simulink model "simulacija"  (Simulink 10.2)
settings: Solver=ode45  StartTime=0.0  StopTime=150  RelTol=1e-3
libraries: simulink x3, fuzblock x1
settings Model: Creator=Aleksandar Markovic  LastModifiedBy=zelimir
settings DataIOCC: SaveFormat=StructureWithTime  SignalLoggingSaveFormat=Dataset
settings DebuggingCC: UnderspecifiedInitializationDetection=Simplified  MergeDetectMultiDrivingBlocksExec=error  SFUnexpectedBacktrackingDiag=error  SFNoUnconditionalDefaultTransitionDiag=error
settings HardwareCC: ProdBitPerPointer=64  ProdLargestAtomicFloat=Float  ProdIntDivRoundTo=Zero  ProdEndianess=LittleEndian  ProdHWDeviceType=Specified
settings GRTTargetCC: TargetLangStandard=C99 (ISO)
settings ConfigComp: CovMetricSettings=dwe  CovSaveCumulativeToWorkspaceVar=off  CovSaveSingleToWorkspaceVar=off  CovExternalEMLEnable=on

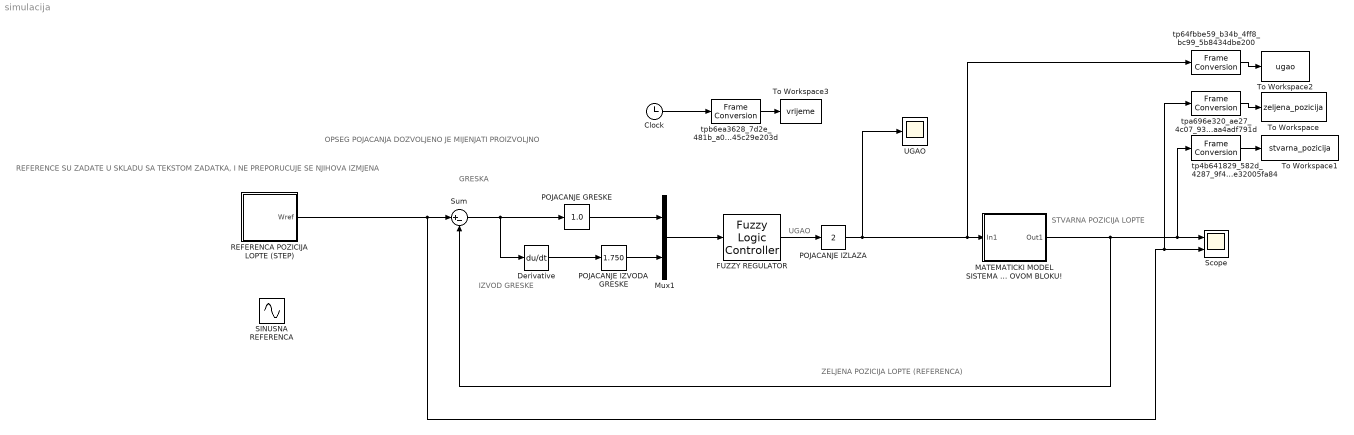
== system simulacija ==
  note: REFERENCE SU ZADATE U SKLADU SA TEKSTOM ZADATKA, I NE PREPORUCUJE SE NJIHOVA IZMJENA
  note: OPSEG POJACANJA DOZVOLJENO JE MIJENJATI PROIZVOLJNO
  note: ZELJENA POZICIJA LOPTE (REFERENCA)
  note: UGAO
  note: GRESKA
  note: IZVOD GRESKE
  note: STVARNA POZICIJA LOPTE
  Clock : Clock
  Derivative : Derivative
  FUZZY REGULATOR : fuzblock/Fuzzy Logic  Controller  FIS='Regulator.fis'  OutputSampleNumber=101  DataType=double  FuzzifiedInputs=off  RuleFiringStrengths=off  RuleOutputs=off  AggregatedOutputs=off  SimulateUsing=Interpreted execution  OutOfRangeInputValueMessage=warning  NoRuleFiredMessage=warning  EmptyOutputFuzzySetMessage=warning
  "MATEMATICKI MODEL SISTEMA OSIM POCETNE POZICIJE,  NE MIJENJATI NISTA DRUGO U OVOM BLOKU!" : Subsystem  mask{pocetna_pozicija=0}
      mask prompts: pocetna_pozicija "POCETNA POZICIJA [0, 1]"
  Mux1 : Mux  Inputs=2
  POJACANJE GRESKE : simulink/Math Operations/Slider Gain  gain=1.0  low=0  high=2
  POJACANJE IZLAZA : simulink/Math Operations/Slider Gain  gain=2  low=0  high=100
  POJACANJE IZVODA GRESKE : simulink/Math Operations/Slider Gain  gain=1.750  low=0  high=5
  REFERENCA POZICIJA LOPTE (STEP) : Subsystem
  SINUSNA REFERENCA : Sin  Amplitude=0.3  Bias=0.5  Frequency=0.2  SampleTime=0
  Scope : Scope  NumInputPorts=2
  Sum : Sum  Inputs=|+-
  To Workspace : ToWorkspace  VariableName=zeljena_pozicija  SampleTime=-1
  To Workspace1 : ToWorkspace  VariableName=stvarna_pozicija  SampleTime=-1
  To Workspace2 : ToWorkspace  VariableName=ugao  SampleTime=-1
  To Workspace3 : ToWorkspace  VariableName=vrijeme  SampleTime=-1
  UGAO : Scope
  tp4b641829_582d_4287_9f41_02e32005fa84 : FrameConversion  OutFrame=Sample-based
  tp64fbbe59_b34b_4ff8_bc99_5b8434dbe200 : FrameConversion  OutFrame=Sample-based
  tpa696e320_ae27_4c07_93dd_8aaa4adf791d : FrameConversion  OutFrame=Sample-based
  tpb6ea3628_7d2e_481b_a00a_9d45c29e203d : FrameConversion  OutFrame=Sample-based
  wires:
  "MATEMATICKI MODEL SISTEMA OSIM POCETNE POZICIJE,  NE MIJENJATI NISTA DRUGO U OVOM BLOKU!"/1(Out1) -> Scope/1, tp4b641829_582d_4287_9f41_02e32005fa84/1, Sum/2
  FUZZY REGULATOR/1 -> POJACANJE IZLAZA/1
  Sum/1 -> POJACANJE GRESKE/1, Derivative/1
  Mux1/1 -> FUZZY REGULATOR/1
  POJACANJE GRESKE/1 -> Mux1/1
  Derivative/1 -> POJACANJE IZVODA GRESKE/1
  POJACANJE IZVODA GRESKE/1 -> Mux1/2
  POJACANJE IZLAZA/1 -> tp64fbbe59_b34b_4ff8_bc99_5b8434dbe200/1, "MATEMATICKI MODEL SISTEMA OSIM POCETNE POZICIJE,  NE MIJENJATI NISTA DRUGO U OVOM BLOKU!"/1(In1), UGAO/1
  tpa696e320_ae27_4c07_93dd_8aaa4adf791d/1 -> To Workspace/1
  tp4b641829_582d_4287_9f41_02e32005fa84/1 -> To Workspace1/1
  tp64fbbe59_b34b_4ff8_bc99_5b8434dbe200/1 -> To Workspace2/1
  Clock/1 -> tpb6ea3628_7d2e_481b_a00a_9d45c29e203d/1
  tpb6ea3628_7d2e_481b_a00a_9d45c29e203d/1 -> To Workspace3/1
  REFERENCA POZICIJA LOPTE (STEP)/1(Wref) -> tpa696e320_ae27_4c07_93dd_8aaa4adf791d/1, Scope/2, Sum/1

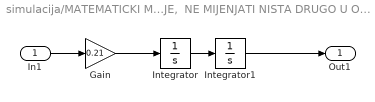
== system simulacija/MATEMATICKI MODEL SISTEMA OSIM POCETNE POZICIJE,  NE MIJENJATI NISTA DRUGO U OVOM BLOKU! ==
  In1 : Inport
  Gain : Gain  Gain=0.21
  Integrator : Integrator  InitialCondition=pocetna_pozicija
  Integrator1 : Integrator  InitialCondition=pocetna_pozicija
  Out1 : Outport
  wires:
  Integrator/1 -> Integrator1/1
  Gain/1 -> Integrator/1
  Integrator1/1 -> Out1/1
  In1/1 -> Gain/1

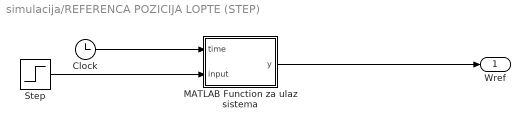
== system simulacija/REFERENCA POZICIJA LOPTE (STEP) ==
  Clock : Clock
  MATLAB Function za ulaz sistema : MATLAB Function  TreatAsAtomicUnit=on
  Step : Step  Time=0  SampleTime=0
  Wref : Outport
  wires:
  Step/1 -> MATLAB Function za ulaz sistema/2(input)
  MATLAB Function za ulaz sistema/1(y) -> Wref/1
  Clock/1 -> MATLAB Function za ulaz sistema/1(time)

== matlab function REFERENCA POZICIJA LOPTE (STEP)/MATLAB Function za ulaz sistema ==
  data: time input double; y output double; input input double
function y = fcn(time, input)
u = input;

if(time >= 0 && time < 35)
    u = u*0.2;
end
if(time >= 35 && time < 60)
    u = u*0.5;
end
if(time >= 60 && time < 85)
    u = 0.7*u;
end
if(time >= 85 && time < 135)
    u = 0.4*u;
end
    
if(time >= 135 && time < 180)
    u = 1*u;
end
y = u;
